simulink model "sim_unconstrained"  (R2016b)
settings: Solver=FixedStepAuto  StartTime=0.0  StopTime=Tf  FixedStep=Ts  RelTol=1e-3
InitFcn:
  | if(~exist('bsol'))
  |    init
  | end
StopFcn:
  | evaluate
values from neighbouring files (symbols this model uses):
  A = blkdiag([0 1;0 0],kron(-diag(omeg.^2),[0 0;1 0])+kron(eye(N),[0 1;0 0]))    [init.m]
  Aa = A(1:2*(Na+1),1:2*(Na+1))    [init.m]
  B = [0;1/J;kron(karr,[0;1])]    [init.m]
  Ba = B(1:2*(Na+1))    [init.m]
  C1a = [1 zeros(1,2*Na+1)]    [init.m]
  C2a = zeros(1,2)    [init.m]
  L = 0.25    [init.m]
  N = length(gamm)    [high_freq_uncert.m]    (also in init.m = 9)
  Na = 1    [init.m]
  X = [0 0.005 0.01 0.015 0.02 0.025 0.03 0.035 0.04 0.045 0.05 0.055 ... (51 elements, 1x51)]    [eigfun.mat]    (also in init.m = 0:h:L)
  z0 = zeros(2*(N+1),1)    [init.m]
  z0a = z0(1:2*(Na+1))    [init.m]
settings Model: Creator=user  LastModifiedBy=user

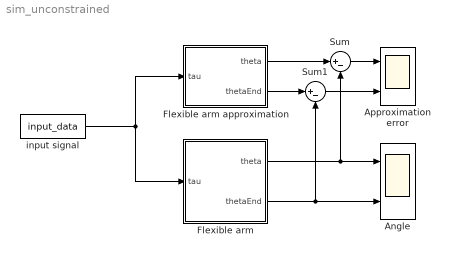
== system sim_unconstrained ==
  Angle : Scope  NumInputPorts=2
  Approximation error : Scope  NumInputPorts=2
  Flexible arm : Subsystem
  Flexible arm approximation : Subsystem
  Sum : Sum  Inputs=|+-
  Sum1 : Sum  Inputs=|+-
  input signal : FromWorkspace  VariableName=input_data  SampleTime=0
  wires:
  Flexible arm/1(theta) -> Sum/2, Angle/1
  input signal/1 -> Flexible arm/1(tau), Flexible arm approximation/1(tau)
  Flexible arm approximation/1(theta) -> Sum/1
  Sum/1 -> Approximation error/1
  Flexible arm/2(thetaEnd) -> Sum1/2, Angle/2
  Flexible arm approximation/2(thetaEnd) -> Sum1/1
  Sum1/1 -> Approximation error/2

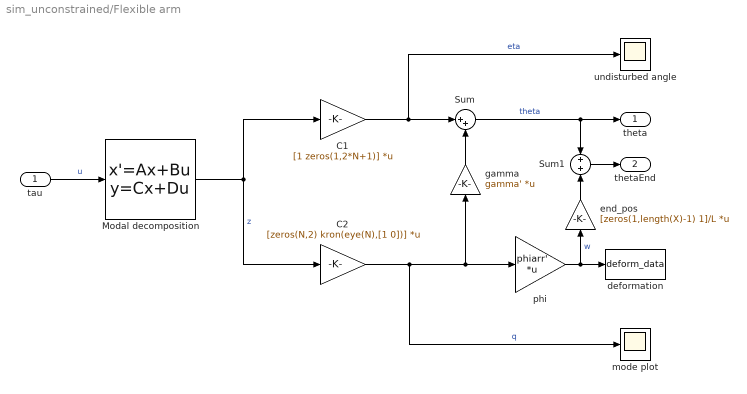
== system sim_unconstrained/Flexible arm ==
  tau : Inport
  C1 : Gain  Gain=[1 zeros(1,2*N+1)]  Multiplication=Matrix(K*u) (u vector)
  C2 : Gain  Gain=[zeros(N,2) kron(eye(N),[1 0])]  Multiplication=Matrix(K*u) (u vector)
  Modal decomposition : StateSpace  A=A  B=B  C=eye(2*(N+1))  D=zeros(2*(N+1),1)  X0=z0
  Sum : Sum  Inputs=|++
  Sum1 : Sum
  deformation : ToWorkspace  VariableName=deform_data  SaveFormat=Structure With Time  SampleTime=-1
  end_pos : Gain  Gain=[zeros(1,length(X)-1) 1]/L  Multiplication=Matrix(K*u)
  gamma : Gain  Gain=gamma'  Multiplication=Matrix(K*u)
  mode plot : Scope
  phi : Gain  Gain=phiarr'  Multiplication=Matrix(K*u)
  undisturbed angle : Scope
  theta : Outport
  thetaEnd : Outport  Port=2
  wires:
  tau/1 -> Modal decomposition/1  "u"
  Modal decomposition/1 -> C1/1, C2/1  "z"
  C1/1 -> undisturbed angle/1, Sum/1  "eta"
  C2/1 -> mode plot/1, phi/1, gamma/1  "q"
  gamma/1 -> Sum/2
  Sum/1 -> Sum1/1, theta/1  "theta"
  phi/1 -> end_pos/1, deformation/1  "w"
  Sum1/1 -> thetaEnd/1
  end_pos/1 -> Sum1/2

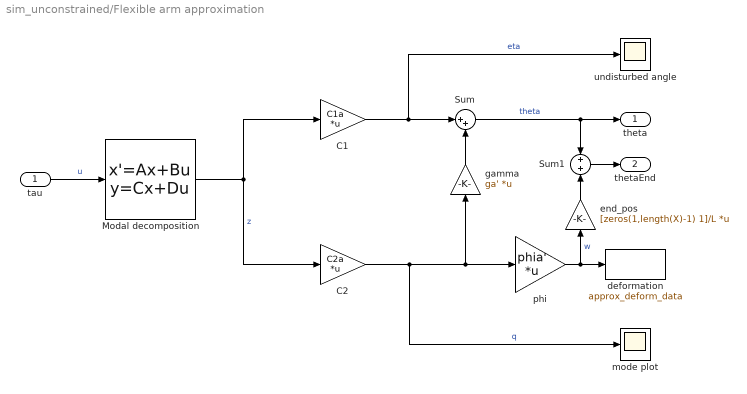
== system sim_unconstrained/Flexible arm approximation ==
  tau : Inport
  C1 : Gain  Gain=C1a  Multiplication=Matrix(K*u) (u vector)
  C2 : Gain  Gain=C2a  Multiplication=Matrix(K*u) (u vector)
  Modal decomposition : StateSpace  A=Aa  B=Ba  C=eye(2*(Na+1))  D=zeros(2*(Na+1),1)  X0=z0a
  Sum : Sum  Inputs=|++
  Sum1 : Sum
  deformation : ToWorkspace  VariableName=approx_deform_data  SaveFormat=Structure With Time  SampleTime=-1
  end_pos : Gain  Gain=[zeros(1,length(X)-1) 1]/L  Multiplication=Matrix(K*u)
  gamma : Gain  Gain=ga'  Multiplication=Matrix(K*u)
  mode plot : Scope
  phi : Gain  Gain=phia'  Multiplication=Matrix(K*u)
  undisturbed angle : Scope
  theta : Outport
  thetaEnd : Outport  Port=2
  wires:
  tau/1 -> Modal decomposition/1  "u"
  Modal decomposition/1 -> C1/1, C2/1  "z"
  C1/1 -> undisturbed angle/1, Sum/1  "eta"
  C2/1 -> mode plot/1, phi/1, gamma/1  "q"
  gamma/1 -> Sum/2
  Sum/1 -> Sum1/1, theta/1  "theta"
  phi/1 -> end_pos/1, deformation/1  "w"
  Sum1/1 -> thetaEnd/1
  end_pos/1 -> Sum1/2
